simulink model "sim_Start_2021b"  (R2022a)
settings: Solver=FixedStepDiscrete  StartTime=0.0  StopTime=30  FixedStep=0.01  RelTol=1e-3
values from neighbouring files (symbols this model uses):
  ticksPerRot = 20    [robotParameters.m]
  wheelR = 0.031    [robotParameters.m]
undefined symbols (not defined in the file or in its folder): InputPWM, WheelSpeed
libraries: mobileRoboticsTrainingLib x6, simulink x2
settings Model: Creator=Boitumelo  LastModifiedBy=heath
settings DebuggingCC: UnconnectedInputMsg=warning  UnconnectedOutputMsg=warning  UnconnectedLineMsg=warning
settings RTWCC: DLArmComputeVersion=19.05

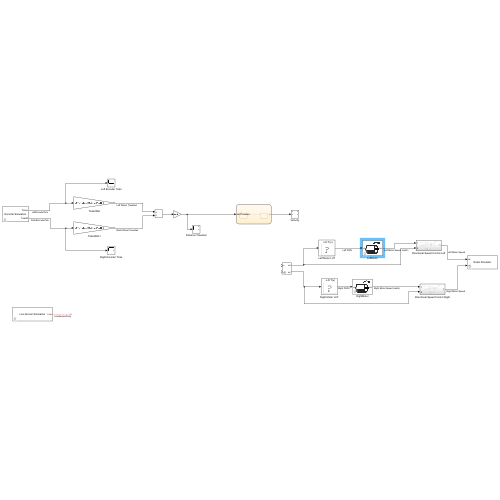
[thumbnail: Simulink's stored preview of the top-level diagram]
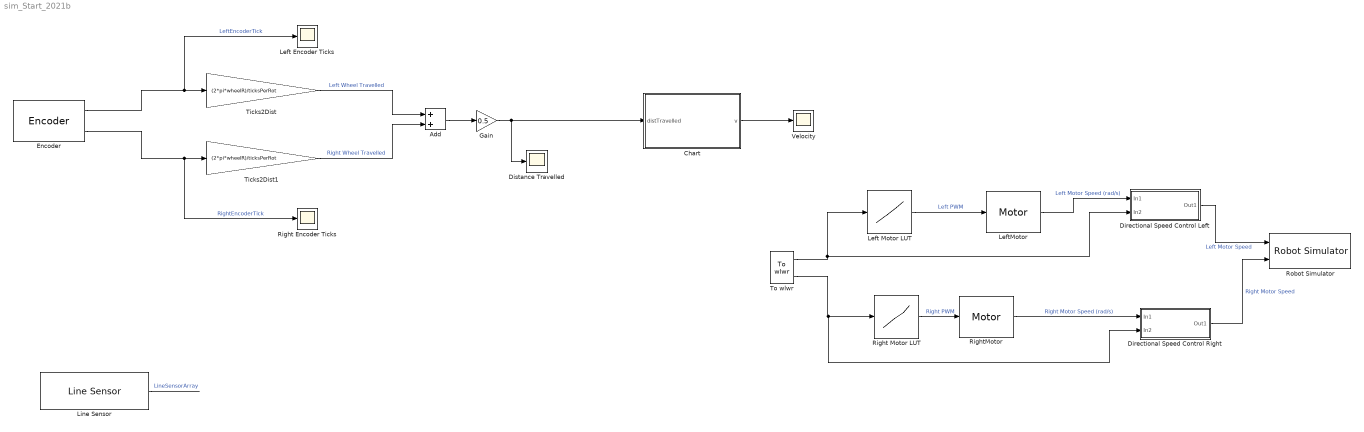
== system sim_Start_2021b ==
  Add : Sum
  Chart : Stateflow chart  TreatAsAtomicUnit=on
  Directional Speed Control Left : Subsystem
  Directional Speed Control Right : Subsystem
  Distance Travelled : Scope
  Encoder : mobileRoboticsTrainingLib/Encoder  axleLength=axleLength  wheelR=wheelR  ticksPerRot=ticksPerRot
      settings: SourceProductName=Mobile Robotics Training Library
  Gain : Gain  Gain=0.5
  Left Encoder Ticks : Scope
  Left Motor LUT : Lookup_n-D  NumberOfTableDimensions=1  BreakpointsForDimension1=WheelSpeed  Table=InputPWM  InterpMethod=Nearest  ExtrapMethod=Clip  InternalRulePriority=Speed  RndMeth=Simplest
  LeftMotor : mobileRoboticsTrainingLib/Motor  motorPlant=wheelMotorModel  sensorType=Speed
      settings: SourceProductName=Mobile Robotics Training Library
  Line Sensor : mobileRoboticsTrainingLib/Line Sensor  mapVariable=mapForSim  envVal=1  lineVal=0  sensOff=[0 0; 0 0; 0 0; 0 0]
      settings: SourceProductName=Mobile Robotics Training Library
  Right Encoder Ticks : Scope
  Right Motor LUT : Lookup_n-D  NumberOfTableDimensions=1  BreakpointsForDimension1=WheelSpeed  Table=InputPWM  InterpMethod=Nearest  ExtrapMethod=Clip  InternalRulePriority=Speed  RndMeth=Simplest
  RightMotor : mobileRoboticsTrainingLib/Motor  motorPlant=wheelMotorModel  sensorType=Speed
      settings: SourceProductName=Mobile Robotics Training Library
  Robot Simulator : mobileRoboticsTrainingLib/Robot Simulator  Priority=99  mapVar=mapForSim  startX=0.2126  startY=0.077048  startTheta=0  axleLength=axleLength  wheelR=wheelR
  Ticks2Dist : Gain  Gain=(2*pi*wheelR)/ticksPerRot
  Ticks2Dist1 : Gain  Gain=(2*pi*wheelR)/ticksPerRot
  To wlwr : mobileRoboticsTrainingLib/To wlwr  axleLength=0.1  wheelR=0.05
  Velocity : Scope
  wires:
  Directional Speed Control Left/1(Out1) -> Robot Simulator/1  "Left Motor Speed"
  Right Motor LUT/1 -> RightMotor/1  "Right PWM"
  Left Motor LUT/1 -> LeftMotor/1  "Left PWM"
  Encoder/1 -> Ticks2Dist/1, Left Encoder Ticks/1  "LeftEncoderTick"
  Encoder/2 -> Ticks2Dist1/1, Right Encoder Ticks/1  "RightEncoderTick"
  To wlwr/1 -> Directional Speed Control Left/2(In2), Left Motor LUT/1
  To wlwr/2 -> Directional Speed Control Right/2(In2), Right Motor LUT/1
  Line Sensor/1 -> ?  "LineSensorArray"
  RightMotor/1 -> Directional Speed Control Right/1(In1)  "Right Motor Speed (rad/s)"
  LeftMotor/1 -> Directional Speed Control Left/1(In1)  "Left Motor Speed (rad/s)"
  Directional Speed Control Right/1(Out1) -> Robot Simulator/2  "Right Motor Speed"
  Add/1 -> Gain/1
  Chart/1(v) -> Velocity/1
  Ticks2Dist/1 -> Add/1  "Left Wheel Travelled"
  Ticks2Dist1/1 -> Add/2  "Right Wheel Travelled"
  Gain/1 -> Chart/1(distTravelled), Distance Travelled/1

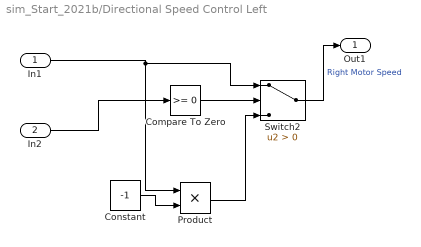
== system sim_Start_2021b/Directional Speed Control Left ==
  In1 : Inport
  In2 : Inport  Port=2
  Compare To Zero : simulink/Logic and Bit Operations/Compare To Zero  relop=>=  OutDataTypeStr=boolean
  Constant : Constant  Value=-1
  Product : Product
  Switch2 : Switch  Criteria=u2 > Threshold  SaturateOnIntegerOverflow=off  InputSameDT=off
  Out1 : Outport
  wires:
  Compare To Zero/1 -> Switch2/2
  In1/1 -> Switch2/1, Product/1
  Constant/1 -> Product/2
  Product/1 -> Switch2/3
  In2/1 -> Compare To Zero/1
  Switch2/1 -> Out1/1  "Right Motor Speed"

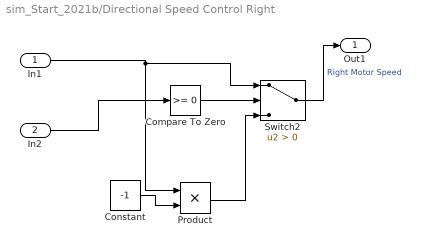
== system sim_Start_2021b/Directional Speed Control Right ==
  In1 : Inport
  In2 : Inport  Port=2
  Compare To Zero : simulink/Logic and Bit Operations/Compare To Zero  relop=>=  OutDataTypeStr=boolean
  Constant : Constant  Value=-1
  Product : Product
  Switch2 : Switch  Criteria=u2 > Threshold  SaturateOnIntegerOverflow=off  InputSameDT=off
  Out1 : Outport
  wires:
  Compare To Zero/1 -> Switch2/2
  In1/1 -> Switch2/1, Product/1
  Constant/1 -> Product/2
  Product/1 -> Switch2/3
  In2/1 -> Compare To Zero/1
  Switch2/1 -> Out1/1  "Right Motor Speed"

== stateflow chart sim_Start_2021b/Chart ==
  state MoveForward
    entry:
    v = 0.1;
  state Stop
    entry:
    v = 0;
  (default) -> MoveForward : %Start
  MoveForward -> Stop : [distTravelled >=1]
  data: distTravelled input; v output
